simulink model "ver1_3DOF_draft2"  (R2023b)
settings: Solver=FixedStepAuto  StartTime=current_time  StopTime=40  RelTol=1e-3
values from neighbouring files (symbols this model uses):
  current_height = 0    [wrapper_for_simulink.m]
  current_pitch = 0    [wrapper_for_simulink.m]
  current_vel = 0    [wrapper_for_simulink.m]
undefined symbols (not defined in the file or in its folder): HDBK, Light, magnitude, MIL, STD
libraries: aerolibwind2 x3, aerolibasang x2, aerolibadyn x1, aerolibatmos2 x1
settings Model: Creator=User  LastModifiedBy=User
settings DataIOCC: ReturnWorkspaceOutputsName=tp3ca22a37_fc90_43f8_8ebe_8c0e39ad763e
settings DebuggingCC: AlgebraicLoopMsg=none  ArtificialAlgebraicLoopMsg=none

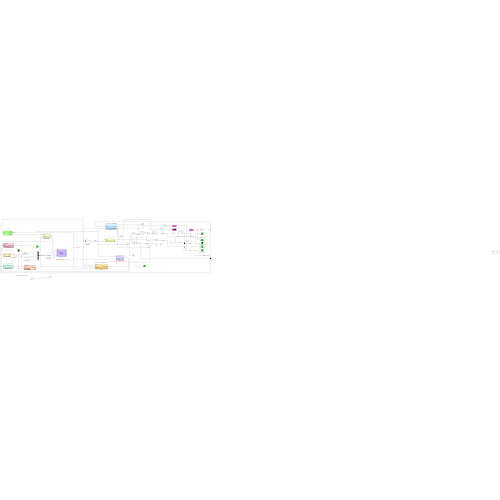
[thumbnail: Simulink's stored preview of the top-level diagram]
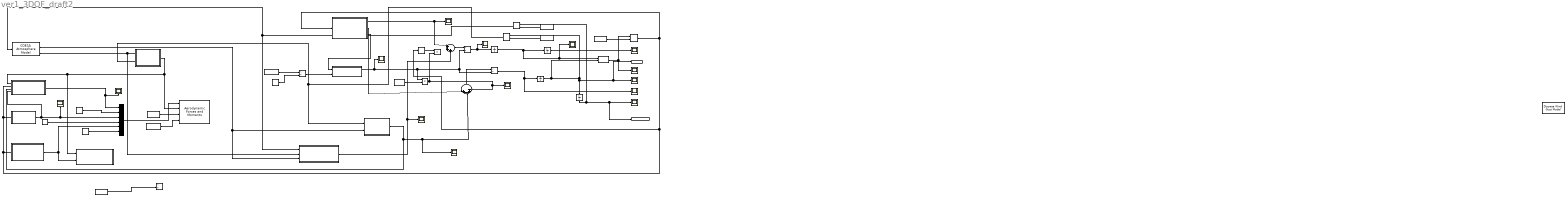
== system ver1_3DOF_draft2 ==
  note: pitch damping moment: see pg 44 of OR doc
  note: ignore everything after v = 0
  note: need to figure out how the wind parameters here
  note: why is this so high???
  note: drag is too high rn at high mach, will need to wait for better drag curve
  note: future me issue :), doesn't have much impact on the sim
      | (Take into consideration later)
  " m(t)" : Subsystem
  "Aerodynamic Forces and Moments " : aerolibadyn/Aerodynamic Forces and Moments   inputAxes=Body  outputForceAxes=Body  outputMomentAxes=Body  S=0.016513  b=2.91  cbar=0.145
  Atan2 : Trigonometry  Operator=atan2
  Axial force coefficient : Subsystem
  CG rocket : Constant  Value=[0 0 1.16]  VectorParams1D=off
  COESA Atmosphere Model : aerolibatmos2/COESA Atmosphere Model  units=Metric (MKS)  spec=MIL-STD-210C  model=Profile  profile_var=Low temperature  profile_percent=10%  profile_alt=5 km (16404 ft)  envelope_var=High temperature  envelope_percent=1%  action=Warning
  CP rocket : Constant  Value=[0 0 0.95]  VectorParams1D=off
  Delay1 : Delay  DelayLength=1  InitialConditionSource=Input port
      settings: InputPortMap=u0,p4
  Delay2 : Delay  DelayLength=1  InitialConditionSource=Input port
      settings: InputPortMap=u0,p4
  Delay3 : Delay  DelayLength=1  InitialConditionSource=Input port
      settings: InputPortMap=u0,p4
  Discrete Wind Gust Model : aerolibwind2/Discrete Wind Gust Model  units=Metric (MKS)  Gx=on  Gy=on  Gz=on  t_0=5  d_m=[120 120 80]  v_m=[3.5 3.5 3.0]
  Divide{,1..3} (4 alike) : Product  Inputs=*/
  Dynamic Pressure : Subsystem
  Flight path angle : Scope
  Integrator{,1..3} (4 alike) : Integrator
  Normal Force coefficient : Subsystem
  Pitch moment : Subsystem
  Pitch moment coefficient : Subsystem
  Product1 : Product
  Product2 : Product
  Scope{,1..8} (9 alike) : Scope
  Side force coefficient : Constant  Value=0
  Sin : Trigonometry
  Sum : Sum  Inputs=|+--+-
  Sum1 : Sum  Inputs=|+++
  Vector Concatenate : Concatenate  NumInputs=6
  WIND : Subsystem
  current height : Constant  Value=current_height
  current pitch : Constant  Value=current_pitch
  current velocity : Constant  Value=current_vel
  drag : Subsystem
  gravity g : Constant  Value=9.80665
  horizontal distance : Scope
  moi : Constant  Value=18.065
  propellant mass : Constant  Value=9.4
  roll moment coefficient : Constant  Value=0
  thrust : Subsystem
  total impulse : Constant  Value=20145.7
  vertical acceleration : Scope
  vertical height : Scope
  vertical velocity in earth ref : Scope
  yaw moment coefficient : Constant  Value=0
  Out1 : Outport  SignalName=height
  Out2 : Outport  Port=2  SignalName=velocity
  wires:
  Integrator1/1 -> Atan2/2, Integrator/1, Out2/1, vertical velocity in earth ref/1, Delay2/1  "velocity"
  CG rocket/1 -> "Aerodynamic Forces and Moments "/3
  CP rocket/1 -> "Aerodynamic Forces and Moments "/4
  COESA Atmosphere Model/2 -> WIND/3(speed of sound), drag/2(speed of sound)  "speed of sound"
  Sum/1 -> Divide1/1
  thrust/2(vertical thrust) -> Sum/1
  Delay1/1 -> Sin/1, Axial force coefficient/2(pitch angle), Normal Force coefficient/1(pitch angle), Pitch moment coefficient/1(pitch angle), thrust/1(pitch angle)
  drag/1(Drag Force) -> Axial force coefficient/3(Drag Force), Scope2/1, Sum/3
  Dynamic Pressure/1(qbar) -> "Aerodynamic Forces and Moments "/2, Pitch moment/1(dynammic pressure), Axial force coefficient/1(dynammic pressure)
  Side force coefficient/1 -> Vector Concatenate/2
  roll moment coefficient/1 -> Vector Concatenate/4
  Normal Force coefficient/1(Normal) -> Axial force coefficient/4(Normal Force coefficient), Vector Concatenate/3, Scope1/1  "Normal Force coefficient"
  Pitch moment coefficient/1(pitch moment coefficient) -> Pitch moment/2(pitch moment coefficient), Vector Concatenate/5
  yaw moment coefficient/1 -> Vector Concatenate/6
  Delay2/1 -> drag/1(velocity vector), Dynamic Pressure/2(velocity signal)
  current velocity/1 -> Delay2/2
  current height/1 -> Delay3/2
  current pitch/1 -> Delay1/2
  COESA Atmosphere Model/4 -> WIND/2(In2), Dynamic Pressure/1(Air Density)
  " m(t)"/1(m(t)) -> Scope6/1, Product1/1, Divide1/2, Divide2/2
  thrust/3(magnitude of T) -> " m(t)"/1(thrust)
  Integrator/1 -> Delay3/1, Out1/1, vertical height/1  "height"
  gravity g/1 -> Product1/2
  Vector Concatenate/1 -> "Aerodynamic Forces and Moments "/1  "aerodynamic coefficients"
  Axial force coefficient/1("axial force coefficient ") -> Scope4/1, Vector Concatenate/1
  total impulse/1 -> Divide/1
  propellant mass/1 -> Divide/2
  Divide/1 -> " m(t)"/2(exhaust velocity)
  Divide1/1 -> vertical acceleration/1, Integrator1/1  "vertical accel"
  Atan2/1 -> Delay1/1, Flight path angle/1
  Delay3/1 -> WIND/1(Altitude), COESA Atmosphere Model/1
  Sum1/1 -> Divide2/1  "Fx"
  WIND/1(wind force u direction) -> Scope3/1, Sum1/3
  Integrator2/1 -> Scope/1, Atan2/1, Integrator3/1  "horizontal vel"
  Integrator3/1 -> horizontal distance/1
  Divide2/1 -> Scope8/1, Integrator2/1  "horizontal accel"
  Product1/1 -> Scope5/1, Sum/5, Product2/2  "gravitational"
  Sin/1 -> Product2/1
  thrust/1(horizontal thrust) -> Sum1/1, Scope7/1
  moi/1 -> Divide3/2

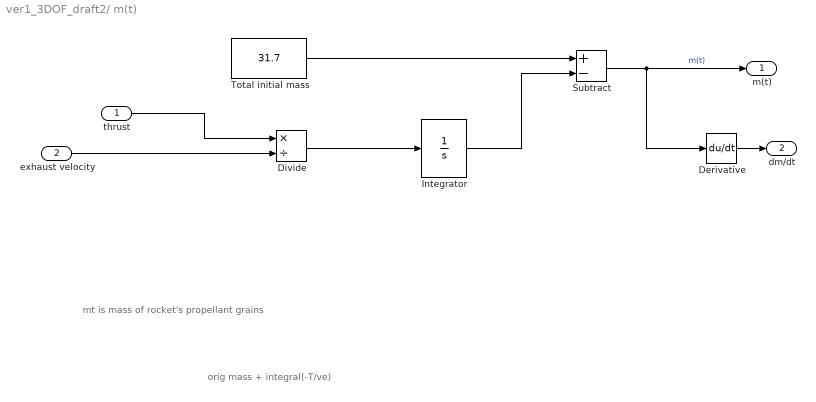
== system ver1_3DOF_draft2/ m(t) ==
  note: orig mass + integral(-T/ve)
  note: mt is mass of rocket's propellant grains
  thrust : Inport
  exhaust velocity : Inport  Port=2
  Derivative : Derivative
  Divide : Product  Inputs=*/
  Integrator : Integrator
  Subtract : Sum  Inputs=+-
  Total initial mass : Constant  Value=31.7
  m(t) : Outport
  dm/dt : Outport  Port=2
  wires:
  Total initial mass/1 -> Subtract/1
  Subtract/1 -> Derivative/1, m(t)/1  "m(t)"
  thrust/1 -> Divide/1
  exhaust velocity/1 -> Divide/2
  Divide/1 -> Integrator/1
  Integrator/1 -> Subtract/2
  Derivative/1 -> dm/dt/1

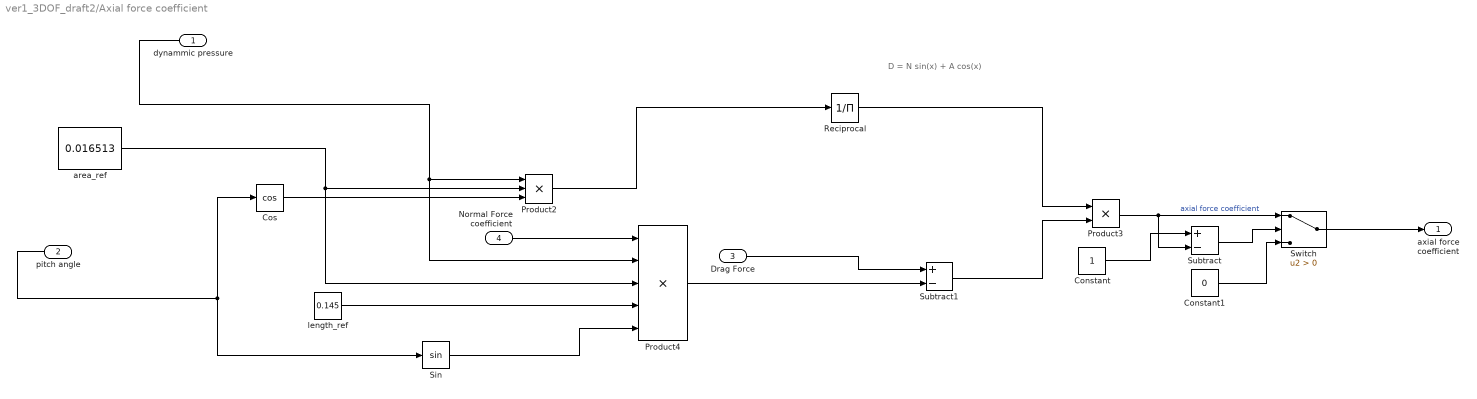
== system ver1_3DOF_draft2/Axial force coefficient ==
  note: D = N sin(x) + A cos(x)
  dynammic pressure : Inport
  pitch angle : Inport  Port=2
  Drag Force : Inport  Port=3
  Normal Force coefficient : Inport  Port=4
  Constant : Constant
  Constant1 : Constant  Value=0
  Cos : Trigonometry  Operator=cos
  Product2 : Product  Inputs=3
  Product3 : Product
  Product4 : Product  Inputs=5
  Reciprocal : Product  Inputs=/
  Sin : Trigonometry
  Subtract : Sum  Inputs=+-
  Subtract1 : Sum  Inputs=+-
  Switch : Switch  Criteria=u2 > Threshold  SaturateOnIntegerOverflow=off  InputSameDT=off
  area_ref : Constant  Value=0.016513
  length_ref : Constant  Value=0.145
  "axial force coefficient " : Outport
  wires:
  Sin/1 -> Product4/5
  pitch angle/1 -> Sin/1, Cos/1
  Normal Force coefficient/1 -> Product4/1
  dynammic pressure/1 -> Product4/2, Product2/1
  area_ref/1 -> Product2/2, Product4/3
  Cos/1 -> Product2/3
  length_ref/1 -> Product4/4
  Product4/1 -> Subtract1/2
  Product3/1 -> Subtract/2, Switch/1  "axial force coefficient"
  Subtract1/1 -> Product3/2
  Drag Force/1 -> Subtract1/1
  Product2/1 -> Reciprocal/1
  Reciprocal/1 -> Product3/1
  Switch/1 -> "axial force coefficient "/1
  Constant/1 -> Subtract/1
  Subtract/1 -> Switch/2
  Constant1/1 -> Switch/3

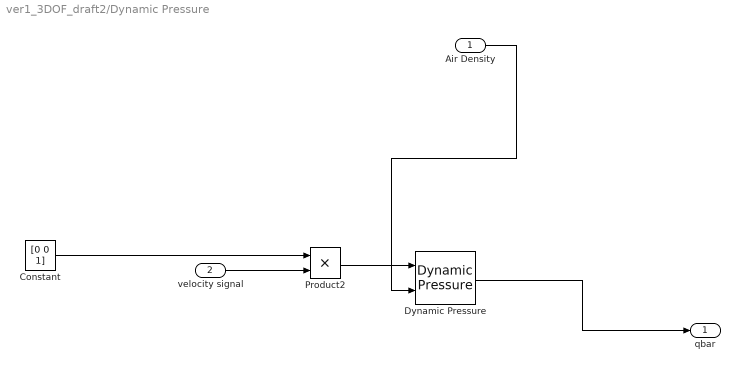
== system ver1_3DOF_draft2/Dynamic Pressure ==
  Air Density : Inport
  velocity signal : Inport  Port=2
  Constant : Constant  Value=[0 0 1]  VectorParams1D=off
  Dynamic Pressure : aerolibasang/Dynamic Pressure
  Product2 : Product
  qbar : Outport
  wires:
  Product2/1 -> Dynamic Pressure/1
  Constant/1 -> Product2/1
  Dynamic Pressure/1 -> qbar/1
  Air Density/1 -> Dynamic Pressure/2
  velocity signal/1 -> Product2/2

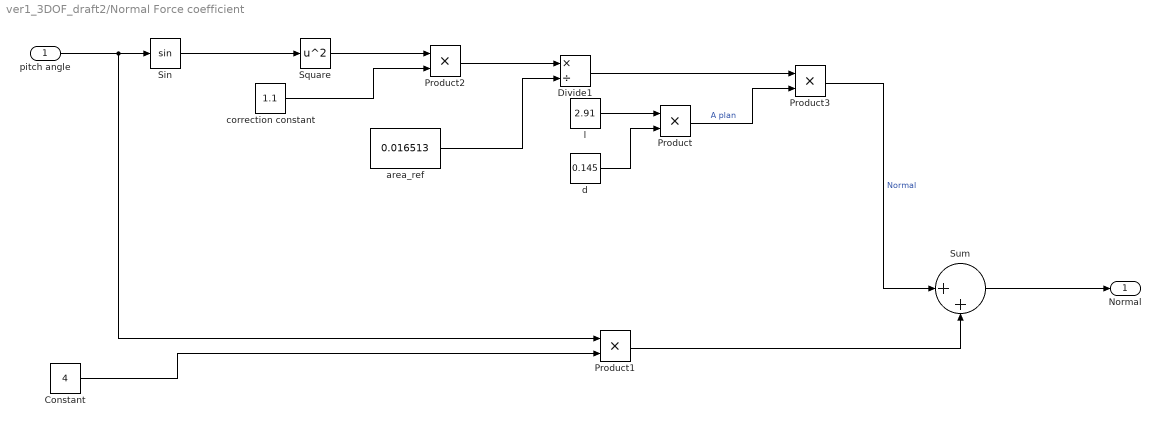
== system ver1_3DOF_draft2/Normal Force coefficient ==
  pitch angle : Inport
  Constant : Constant  Value=4
  Divide1 : Product  Inputs=*/
  Product{,1..3} (4 alike) : Product
  Sin : Trigonometry
  Square : Math  Operator=square
  Sum : Sum  Inputs=|++
  area_ref : Constant  Value=0.016513
  correction constant : Constant  Value=1.1
  d : Constant  Value=0.145
  l : Constant  Value=2.91
  Normal : Outport
  wires:
  pitch angle/1 -> Product1/1, Sin/1
  correction constant/1 -> Product2/2
  Product2/1 -> Divide1/1
  area_ref/1 -> Divide1/2
  Divide1/1 -> Product3/1
  Sin/1 -> Square/1
  Square/1 -> Product2/1
  Product/1 -> Product3/2  "A plan"
  l/1 -> Product/1
  d/1 -> Product/2
  Constant/1 -> Product1/2
  Product1/1 -> Sum/2
  Product3/1 -> Sum/1  "Normal"
  Sum/1 -> Normal/1

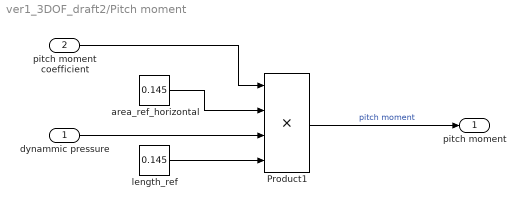
== system ver1_3DOF_draft2/Pitch moment ==
  dynammic pressure : Inport
  pitch moment coefficient : Inport  Port=2
  Product1 : Product  Inputs=4
  area_ref_horizontal : Constant  Value=0.145
  length_ref : Constant  Value=0.145
  pitch moment : Outport
  wires:
  area_ref_horizontal/1 -> Product1/2
  Product1/1 -> pitch moment/1  "pitch moment"
  length_ref/1 -> Product1/4
  dynammic pressure/1 -> Product1/3
  pitch moment coefficient/1 -> Product1/1

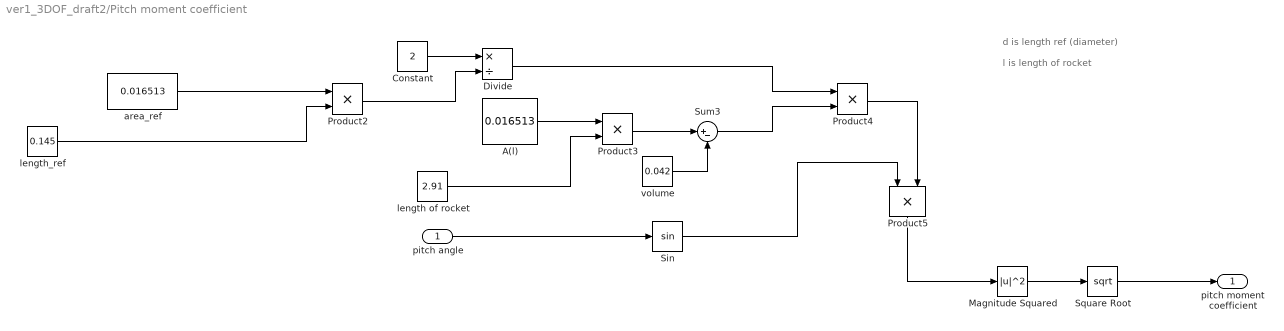
== system ver1_3DOF_draft2/Pitch moment coefficient ==
  note: l is length of rocket
  note: d is length ref (diameter)
  pitch angle : Inport
  A(l) : Constant  Value=0.016513
  Constant : Constant  Value=2
  Divide : Product  Inputs=*/
  Magnitude Squared : Math  Operator=magnitude^2
  Product{2..5} (4 alike) : Product
  Sin : Trigonometry
  Square Root : Sqrt
  Sum3 : Sum  Inputs=|+-
  area_ref : Constant  Value=0.016513
  length of rocket : Constant  Value=2.91
  length_ref : Constant  Value=0.145
  volume : Constant  Value=0.042
  pitch moment coefficient : Outport
  wires:
  length_ref/1 -> Product2/2
  Product2/1 -> Divide/2
  A(l)/1 -> Product3/1
  Product4/1 -> Product5/2
  Product5/1 -> Magnitude Squared/1
  area_ref/1 -> Product2/1
  Product3/1 -> Sum3/1
  Divide/1 -> Product4/1
  volume/1 -> Sum3/2
  Constant/1 -> Divide/1
  pitch angle/1 -> Sin/1
  Sum3/1 -> Product4/2
  Sin/1 -> Product5/1
  length of rocket/1 -> Product3/2
  Magnitude Squared/1 -> Square Root/1
  Square Root/1 -> pitch moment coefficient/1

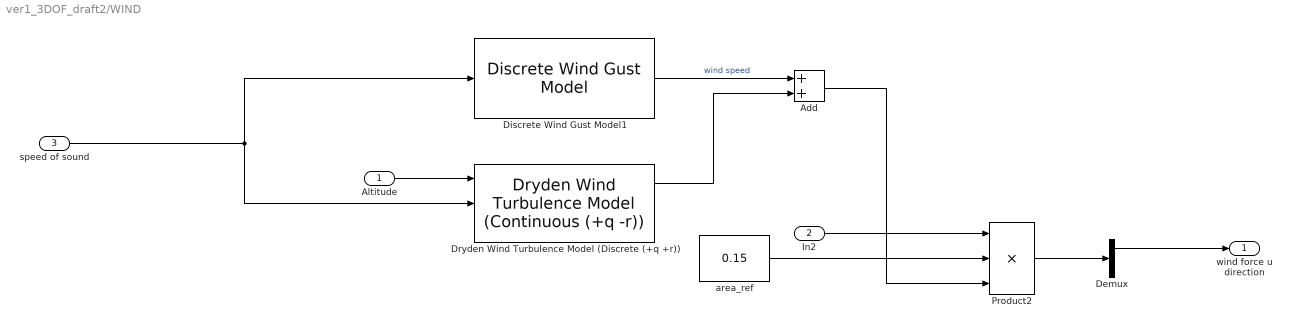
== system ver1_3DOF_draft2/WIND ==
  Altitude : Inport
  In2 : Inport  Port=2
  speed of sound : Inport  Port=3
  Add : Sum
  Demux : Demux  Outputs=3
  Discrete Wind Gust Model1 : aerolibwind2/Discrete Wind Gust Model  units=Metric (MKS)  Gx=on  Gy=on  Gz=on  t_0=0  d_m=[50 80 50]  v_m=[1 2 3.0]
  Dryden Wind Turbulence Model (Discrete (+q +r)) : aerolibwind2/Dryden Wind Turbulence Model  (Continuous (+q -r))  units=Metric (MKS)  spec=MIL-HDBK-1797B  model=Discrete Dryden (+q +r)  W20=5  Wdeg=10  TurbProb=10^-2 - Light  L_high=533.4  Wingspan=10  ts=0.1  Seed=[23341 23342 23343 23344]  T_on=on
      settings: LibrarySourceBlock=|
      | aerolibwind2/Dryden Wind Turbulence Model
      | (Discrete (+q +r))
  Product2 : Product  Inputs=3
  area_ref : Constant  Value=0.15
  wind force u direction : Outport
  wires:
  In2/1 -> Product2/1
  area_ref/1 -> Product2/2
  Dryden Wind Turbulence Model (Discrete (+q +r))/1 -> Add/2
  speed of sound/1 -> Discrete Wind Gust Model1/1, Dryden Wind Turbulence Model (Discrete (+q +r))/2
  Product2/1 -> Demux/1
  Altitude/1 -> Dryden Wind Turbulence Model (Discrete (+q +r))/1
  Discrete Wind Gust Model1/1 -> Add/1  "wind speed"
  Add/1 -> Product2/3
  Demux/1 -> wind force u direction/1

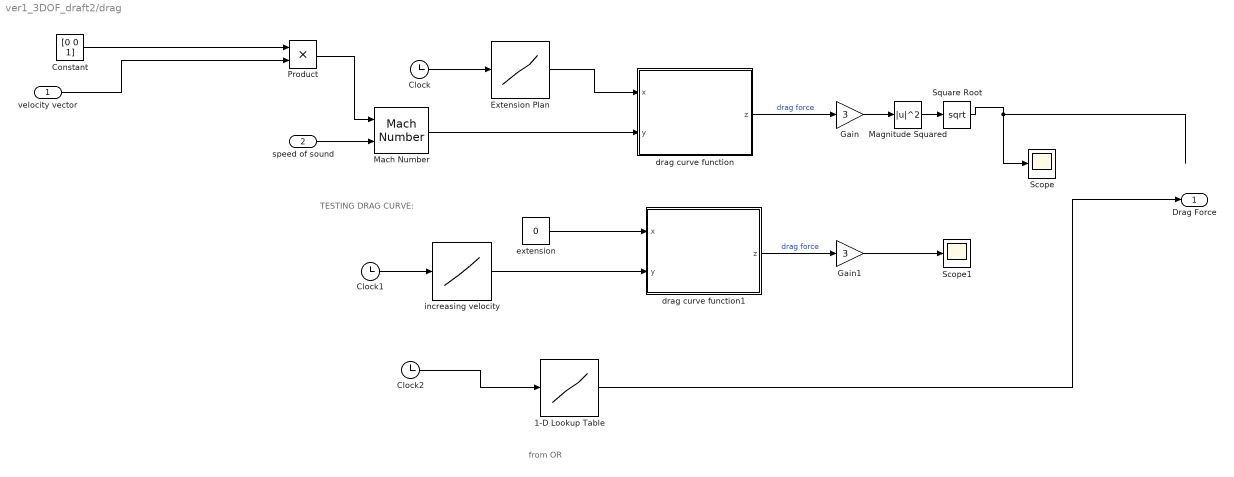
== system ver1_3DOF_draft2/drag ==
  note: from OR
  note: TESTING DRAG CURVE:
  velocity vector : Inport
  speed of sound : Inport  Port=2
  1-D Lookup Table : Lookup_n-D  NumberOfTableDimensions=1  BreakpointsForDimension1=|  Table=|  InternalRulePriority=Speed  RndMeth=Simplest
      BreakpointsForDimension1=|
      | [0.01
      | 0.02
      | 0.03
      | 0.04
      | 0.05
      | 0.06
      | 0.07
      | 0.078
      | 0.085
      | 0.092
      | 0.098
      | 0.104
      | 0.109
      | 0.114
      | 0.121
      | 0.133
      | 0.15
      | 0.175
      | 0.213
      | 0.263
      | 0.313
      | 0.363
      | 0.413
      | 0.463
      | 0.513
      | 0.563
      | 0.613
      | 0.663
      | 0.713
      | 0.763
      | 0.813
      | 0.863
      | 0.913
      | 0.963
      | 1.013
      | 1.063
      | 1.113
      | 1.163
      | 1.213
      | 1.263
      | 1.313
      | 1.363
      | 1.413
      | 1.463
      | 1.513
      | 1.563
      | 1.613
      | 1.663
      | 1.713
      | 1.763
      | 1.813
      | 1.863
      | 1.913
      | 1.963
      | 2.013
      | 2.063
      | 2.113
      | 2.163
      | 2.213
      | 2.263
      | 2.313
      | 2.363
      | 2.413
      | 2.463
      | 2.513
      | 2.563
      | 2.613
      | 2.663
      | 2.713
      | 2.763
      | 2.813
      | 2.863
      | 2.913
      | 2.963
      | 3.013
      | 3.063
      | 3.113
      | 3.163
      | 3.213
      | 3.263
      | 3.313
      | 3.363
      | 3.413
      | 3.463
      | 3.513
      | 3.563
      | 3.594
      | 3.64
      | 3.69
      | 3.74
      | 3.79
      | 3.84
      | 3.89
      | 3.94
      | 3.99
      | 4.04
      | 4.09
      | 4.14
      | 4.19
      | 4.24
      | 4.29
      | 4.34
      | 4.39
      | 4.44
      | 4.49
      | 4.54
      | 4.59
      | 4.64
      | 4.69
      | 4.74
      | 4.79
      | 4.84
      | 4.89
      | 4.94
      | 4.99
      | 5.04
      | 5.09
      | 5.14
      | 5.19
      | 5.24
      | 5.29
      | 5.34
      | 5.39
      | 5.44
      | 5.49
      | 5.54
      | 5.59
      | 5.64
      | 5.69
      | 5.74
      | 5.79
      | 5.84
      | 5.89
      | 5.94
      | 5.99
      | 6.04
      | 6.09
      | 6.14
      | 6.19
      | 6.24
      | 6.29
      | 6.34
      | 6.39
      | 6.44
      | 6.49
      | 6.54
      | 6.59
      | 6.64
      | 6.69
      | 6.74
      | 6.79
      | 6.84
      | 6.89
      | 6.94
      | 6.99
      | 7.04
      | 7.09
      | 7.14
      | 7.19
      | 7.24
      | 7.29
      | 7.34
      | 7.39
      | 7.44
      | 7.49
      | 7.54
      | 7.59
      | 7.64
      | 7.69
      | 7.74
      | 7.79
      | 7.84
      | 7.89
      | 7.94
      | 7.99
      | 8.04
      | 8.09
      | 8.14
      | 8.19
      | 8.24
      | 8.29
      | 8.34
      | 8.39
      | 8.44
      | 8.49
      | 8.54
      | 8.59
      | 8.64
      | 8.69
      | 8.74
      | 8.79
      | 8.84
      | 8.89
      | 8.94
      | 8.99
      | 9.04
      | 9.09
      | 9.14
      | 9.19
      | 9.24
      | 9.29
      | 9.34
      | 9.39
      | 9.44
      | 9.49
      | 9.54
      | 9.59
      | 9.64
      | 9.69
      | 9.74
      | 9.79
      | 9.84
      | 9.89
      | 9.94
      | 9.99
      | 10.04
      | 10.09
      | 10.14
      | 10.19
      | 10.24
      | 10.29
      | 10.34
      | 10.39
      | 10.44
      | 10.49
      | 10.54
      | 10.59
      | 10.64
      | 10.69
      | 10.74
      | 10.79
      | 10.84
      | 10.89
      | 10.94
      | 10.99
      | 11.04
      | 11.09
      | 11.14
      | 11.19
      | 11.24
      | 11.29
      | 11.34
      | 11.39
      | 11.44
      | 11.49
      | 11.54
      | 11.59
      | 11.64
      | 11.69
      | 11.74
      | 11.79
      | 11.84
      | 11.89
      | 11.94
      | 11.99
      | 12.04
      | 12.09
      | 12.14
      | 12.19
      | 12.24
      | 12.29
      | 12.34
      | 12.39
      | 12.44
      | 12.49
      | 12.54
      | 12.59
      | 12.64
      | 12.69
      | 12.74
      | 12.79
      | 12.84
      | 12.89
      | 12.94
      | 12.99
      | 13.04
      | 13.09
      | 13.14
      | 13.19
      | 13.24
      | 13.29
      | 13.34
      | 13.39
      | 13.44
      | 13.49
      | 13.54
      | 13.59
      | 13.64
      | 13.69
      | 13.74
      | 13.79
      | 13.84
      | 13.89
      | 13.94
      | 13.99
      | 14.04
      | 14.09
      | 14.14
      | 14.19
      | 14.24
      | 14.29
      | 14.34
      | 14.39
      | 14.44
      | 14.49
      | 14.54
      | 14.59
      | 14.64
      | 14.69
      | 14.74
      | 14.79
      | 14.84
      | 14.89
      | 14.94
      | 14.99
      | 15.04
      | 15.09
      | 15.14
      | 15.19
      | 15.24
      | 15.29
      | 15.34
      | 15.39
      | 15.44
      | 15.49
      | 15.54
      | 15.59
      | 15.64
      | 15.69
      | 15.74
      | 15.79
      | 15.84
      | 15.89
      | 15.94
      | 15.99
      | 16.04
      | 16.09
      | 16.14
      | 16.19
      | 16.24
      | 16.29
      | 16.34
      | 16.39
      | 16.44
      | 16.49
      | 16.54
      | 16.59
      | 16.64
      | 16.69
      | 16.74
      | 16.79
      | 16.84
      | 16.89
      | 16.94
      | 16.99
      | 17.04
      | 17.09
      | 17.14
      | 17.19
      | 17.24
      | 17.29
      | 17.34
      | 17.39
      | 17.44
      | 17.49
      | 17.54
      | 17.59
      | 17.64
      | 17.69
      | 17.74
      | 17.79
      | 17.84
      | 17.89
      | 17.94
      | 17.99
      | 18.04
      | 18.09
      | 18.14
      | 18.19
      | 18.24
      | 18.29
      | 18.34
      | 18.39
      | 18.44
      | 18.49
      | 18.54
      | 18.59
      | 18.64
      | 18.69
      | 18.74
      | 18.79
      | 18.84
      | 18.89
      | 18.94
      | 18.99
      | 19.04
      | 19.09
      | 19.14
      | 19.19
      | 19.24
      | 19.29
      | 19.34
      | 19.39
      | 19.44
      | 19.49
      | 19.54
      | 19.59
      | 19.64
      | 19.69
      | 19.74
      | 19.79
      | 19.84
      | 19.89
      | 19.94
      | 19.99
      | 20.04
      | 20.09
      | 20.14
      | 20.19
      | 20.24
      | 20.29
      | 20.34
      | 20.39
      | 20.44
      | 20.49
      | 20.54
      | 20.59
      | 20.64
      | 20.69
      | 20.74
      | 20.79
      | 20.84
      | 20.89
      | 20.94
      | 20.99
      | 21.04
      | 21.09
      | 21.14
      | 21.19
      | 21.24
      | 21.29
      | 21.34
      | 21.39
      | 21.44
      | 21.49
      | 21.54
      | 21.59
      | 21.64
      | 21.69
      | 21.74
      | 21.79
      | 21.84
      | 21.89
      | 21.94
      | 21.99
      | 22.04
      | 22.09
      | 22.14
      | 22.19
      | 22.24
      | 22.29
      | 22.34
      | 22.39
      | 22.44
      | 22.49
      | 22.54
      | 22.59
      | 22.64
      | 22.69
      | 22.74
      | 22.79
      | 22.84
      | 22.89
      | 22.94
      | 22.99
      | 23.04
      | 23.09
      | 23.14
      | 23.19
      | 23.24
      | 23.29
      | 23.34
      | 23.39
      | 23.44
      | 23.49
      | 23.54
      | 23.59
      | 23.64
      | 23.69
      | 23.74
      | 23.79
      | 23.84
      | 23.89
      | 23.94
      | 23.99
      | 24.04
      | 24.09
      | 24.14
      | 24.19
      | 24.24
      | 24.29
      | 24.34
      | 24.39
      | 24.44
      | 24.49
      | 24.54
      | 24.59
      | 24.64
      | 24.69
      | 24.74
      | 24.79
      | 24.84
      | 24.89
      | 24.94
      | 24.99
      | 25.04
      | 25.09
      | 25.14
      | 25.19
      | 25.24
      | 25.29
      | 25.34
      | 25.39
      | 25.44
      | 25.49
      | 25.54
      | 25.59
      | 25.64
      | 25.69
      | 25.74
      | 25.79
      | 25.84
      | 25.89
      | 25.94
      | 25.99
      | 26.04
      | 26.09
      | 26.14
      | 26.19
      | 26.24
      | 26.29
      | 26.34
      | 26.39
      | 26.44
      | 26.49
      | 26.54
      | 26.59
      | 26.64
      | 26.69
      | 26.74
      | 26.79
      | 26.84
      | 26.89
      | 26.94
      | 26.99
      | 27.04
      | 27.09
      | 27.14
      | 27.19
      | 27.24
      | 27.29
      | 27.34
      | 27.39
      | 27.44
      | 27.49
      | 27.54
      | 27.59
      | 27.64
      | 27.69
      | 27.74
      | 27.79
      | 27.84
      | 27.89
      | 27.94
      | 27.99
      | 28.04
      | 28.09
      | 28.14
      | 28.19
      | 28.24
      | 28.29
      | 28.34
      | 28.39
      | 28.44
      | 28.49
      | 28.54
      | 28.59
      | 28.64
      | 28.69
      | 28.74
      | 28.79
      | 28.84
      | 28.89
      | 28.94
      | 28.99
      | 29.04
      | 29.09
      | 29.14
      | 29.19
      | 29.24
      | 29.29
      | 29.34
      | 29.39
      | 29.44
      | 29.49
      | 29.54
      | 29.59
      | 29.64
      | 29.69
      | 29.74
      | 29.79
      | 29.84
      | 29.89
      | 29.94
      | 29.99
      | 30.04
      | 30.09
      | 30.14
      | 30.19
      | 30.24
      | 30.29
      | 30.34
      | 30.39
      | 30.44
      | 30.49
      | 30.54
      | 30.59
      | 30.64
      | 30.69
      | 30.74
      | 30.79
      | 30.84
      | 30.89
      | 30.94
      | 30.99
      | 31.04
      | 31.09
      | 31.14
      | 31.19
      | 31.24
      | 31.29
      | 31.34
      | 31.39
      | 31.44
      | 31.49
      | 31.54
      | 31.59
      | 31.64
      | 31.69
      | 31.74
      | 31.79
      | 31.84
      | 31.89
      | 31.94
      | 31.99
      | 32.04
      | 32.09
      | 32.14
      | 32.19
      | 32.24
      | 32.29
      | 32.34
      | 32.39
      | 32.44
      | 32.49
      | 32.54
      | 32.59
      | 32.64
      | 32.69
      | 32.74
      | 32.79
      | 32.84
      | 32.89
      | 32.94
      | 32.99
      | 33.04
      | 33.09
      | 33.14
      | 33.19
      | 33.24
      | 33.29
      | 33.34
      | 33.39
      | 33.44
      | 33.49
      | 33.54
      | 33.59
      | 33.64
      | 33.69
      | 33.74
      | 33.79
      | 33.84
      | 33.89
      | 33.94
      | 33.99
      | 34.04
      | 34.09
      | 34.14
      | 34.19
      | 34.24
      | 34.29
      | 34.34
      | 34.39
      | 34.44
      | 34.49
      | 34.54
      | 34.59
      | 34.64
      | 34.69
      | 34.74
      | 34.79
      | 34.84
      | 34.89
      | 34.94
      | 34.99
      | 35.04
      | 35.09
      | 35.14
      | 35.19
      | 35.24
      | 35.29
      | 35.34
      | 35.39
      | 35.44
      | 35.49
      | 35.54
      | 35.59
      | 35.64
      | 35.69
      | 35.74
      | 35.79
      | 35.84
      | 35.89
      | 35.94
      | 35.99
      | 36.04
      | 36.09
      | 36.14
      | 36.19
      | 36.24
      | 36.29
      | 36.34
      | 36.39
      | 36.44
      | 36.49
      | 36.54
      | 36.59
      | 36.64
      | 36.69
      | 36.74
      | 36.79
      | 36.84
      | 36.89
      | 36.94
      | 36.99
      | 37.04
      | 37.09
      | 37.14
      | 37.19
      | 37.24
      | 37.29
      | 37.34
      | 37.39
      | 37.44
      | 37.49
      | 37.54
      | 37.59
      | 37.64
      | 37.69
      | 37.74
      | 37.79
      | 37.84
      | 37.89
      | 37.94
      | 37.99
      | 38.04
      | 38.09
      | 38.14
      | 38.19
      | 38.24
      | 38.29
      | 38.34
      | 38.39
      | 38.44
      | 38.49
      | 38.54
      | 38.59]
      Table=|
      | [6.45E-04
      | 0.027
      | 0.105
      | 0.212
      | 0.338
      | 0.481
      | 0.642
      | 0.809
      | 0.971
      | 1.131
      | 1.288
      | 1.444
      | 1.597
      | 1.75
      | 1.994
      | 2.391
      | 3.057
      | 4.223
      | 6.343
      | 9.812
      | 14.076
      | 19.157
      | 25.083
      | 31.887
      | 39.581
      | 48.209
      | 57.793
      | 68.372
      | 79.961
      | 92.62
      | 106.378
      | 121.275
      | 137.345
      | 154.63
      | 173.191
      | 193.08
      | 214.392
      | 237.207
      | 261.655
      | 287.921
      | 316.302
      | 347.256
      | 381.815
      | 409.873
      | 439.455
      | 471.847
      | 504.945
      | 536.656
      | 566.911
      | 596.248
      | 625.958
      | 655.947
      | 685.233
      | 714.695
      | 744.391
      | 774.108
      | 803.758
      | 833.016
      | 860.081
      | 886.859
      | 913.355
      | 939.504
      | 965.311
      | 990.775
      | 1014.79
      | 1038.216
      | 1061.179
      | 1083.078
      | 1102.884
      | 1120.561
      | 1136.108
      | 1149.568
      | 1160.938
      | 1170.235
      | 1177.488
      | 1183.267
      | 1188.088
      | 1191.815
      | 1194.392
      | 1195.121
      | 1193.871
      | 1190.726
      | 1185.86
      | 1179.236
      | 1170.729
      | 1161.001
      | 1154.569
      | 1144.059
      | 1132.871
      | 1121.805
      | 1110.852
      | 1100.033
      | 1089.521
      | 1079.134
      | 1068.852
      | 1058.678
      | 1048.611
      | 1038.652
      | 1028.805
      | 1019.068
      | 1009.423
      | 999.893
      | 990.463
      | 981.13
      | 971.899
      | 962.759
      | 953.729
      | 944.789
      | 936.004
      | 927.416
      | 918.919
      | 910.506
      | 902.172
      | 893.931
      | 885.777
      | 877.709
      | 869.72
      | 861.81
      | 853.975
      | 846.226
      | 838.567
      | 830.976
      | 823.465
      | 816.03
      | 808.672
      | 801.382
      | 794.212
      | 787.142
      | 780.028
      | 772.982
      | 766.011
      | 759.116
      | 752.29
      | 745.536
      | 738.855
      | 732.245
      | 725.699
      | 719.217
      | 712.807
      | 706.464
      | 700.185
      | 693.969
      | 687.816
      | 681.728
      | 675.707
      | 669.741
      | 663.905
      | 658.167
      | 652.486
      | 646.859
      | 641.282
      | 635.764
      | 630.3
      | 624.9
      | 619.544
      | 614.241
      | 608.992
      | 603.795
      | 598.657
      | 593.556
      | 588.512
      | 583.512
      | 578.552
      | 573.386
      | 568.273
      | 563.228
      | 558.231
      | 553.307
      | 548.495
      | 543.737
      | 539.025
      | 534.355
      | 529.743
      | 525.18
      | 520.658
      | 516.186
      | 511.757
      | 507.373
      | 503.037
      | 498.737
      | 494.486
      | 490.28
      | 486.111
      | 481.99
      | 477.91
      | 473.87
      | 469.865
      | 465.9
      | 461.977
      | 458.095
      | 454.242
      | 450.495
      | 446.792
      | 443.123
      | 439.484
      | 435.88
      | 432.31
      | 428.774
      | 425.278
      | 421.811
      | 418.376
      | 414.978
      | 411.607
      | 408.266
      | 404.96
      | 401.686
      | 398.438
      | 395.184
      | 391.917
      | 388.683
      | 385.479
      | 382.304
      | 379.158
      | 376.043
      | 372.957
      | 369.901
      | 366.91
      | 363.969
      | 361.048
      | 358.157
      | 355.291
      | 352.456
      | 349.644
      | 346.855
      | 344.099
      | 341.36
      | 338.65
      | 335.964
      | 333.299
      | 330.664
      | 328.054
      | 325.462
      | 322.895
      | 320.352
      | 317.766
      | 315.18
      | 312.617
      | 310.086
      | 307.575
      | 305.085
      | 302.62
      | 300.182
      | 297.762
      | 295.361
      | 293.009
      | 290.699
      | 288.411
      | 286.136
      | 283.879
      | 281.404
      | 278.963
      | 276.543
      | 274.146
      | 271.777
      | 269.437
      | 267.117
      | 264.818
      | 262.54
      | 260.293
      | 258.067
      | 255.864
      | 253.687
      | 251.525
      | 249.382
      | 247.257
      | 245.137
      | 243.044
      | 240.967
      | 238.91
      | 236.877
      | 234.858
      | 232.864
      | 230.889
      | 228.934
      | 226.999
      | 225.106
      | 223.231
      | 221.377
      | 219.541
      | 217.72
      | 215.922
      | 214.198
      | 212.551
      | 210.914
      | 209.292
      | 207.686
      | 206.089
      | 204.505
      | 202.933
      | 201.376
      | 199.835
      | 198.309
      | 196.789
      | 195.285
      | 193.788
      | 192.312
      | 190.846
      | 189.391
      | 187.954
      | 186.284
      | 184.481
      | 182.702
      | 180.957
      | 179.237
      | 177.545
      | 175.875
      | 174.234
      | 172.617
      | 171.026
      | 169.463
      | 167.925
      | 166.408
      | 164.911
      | 163.434
      | 161.976
      | 160.536
      | 159.122
      | 157.722
      | 156.33
      | 154.958
      | 153.603
      | 152.265
      | 150.943
      | 149.637
      | 148.347
      | 147.07
      | 145.809
      | 144.563
      | 143.324
      | 142.099
      | 140.889
      | 139.693
      | 138.51
      | 137.334
      | 136.173
      | 135.023
      | 133.888
      | 132.766
      | 131.657
      | 130.547
      | 129.451
      | 128.372
      | 127.304
      | 126.247
      | 125.195
      | 124.154
      | 123.123
      | 122.107
      | 121.11
      | 120.118
      | 119.136
      | 118.163
      | 117.203
      | 116.246
      | 115.3
      | 114.362
      | 113.435
      | 112.522
      | 111.61
      | 110.707
      | 109.809
      | 108.922
      | 108.045
      | 107.17
      | 106.301
      | 105.443
      | 104.597
      | 103.758
      | 102.918
      | 102.086
      | 101.264
      | 100.452
      | 99.642
      | 98.838
      | 98.046
      | 97.256
      | 96.473
      | 95.697
      | 94.928
      | 94.165
      | 93.408
      | 92.662
      | 91.919
      | 91.176
      | 90.447
      | 89.722
      | 89.003
      | 88.288
      | 87.583
      | 86.88
      | 86.184
      | 85.501
      | 84.824
      | 84.15
      | 83.482
      | 82.819
      | 82.159
      | 81.506
      | 80.86
      | 80.218
      | 79.582
      | 78.951
      | 78.32
      | 77.699
      | 77.079
      | 76.464
      | 75.853
      | 75.25
      | 74.651
      | 74.056
      | 73.465
      | 72.878
      | 72.295
      | 71.719
      | 71.145
      | 70.579
      | 70.018
      | 69.456
      | 68.898
      | 68.348
      | 67.798
      | 67.254
      | 66.718
      | 66.181
      | 65.651
      | 65.123
      | 64.6
      | 64.081
      | 63.566
      | 63.053
      | 62.543
      | 62.038
      | 61.539
      | 61.04
      | 60.547
      | 60.056
      | 59.569
      | 59.088
      | 58.608
      | 58.128
      | 57.659
      | 57.189
      | 56.726
      | 56.269
      | 55.815
      | 55.364
      | 54.915
      | 54.468
      | 54.027
      | 53.587
      | 53.151
      | 52.718
      | 52.29
      | 51.863
      | 51.437
      | 51.015
      | 50.595
      | 50.185
      | 49.77
      | 49.362
      | 48.956
      | 48.555
      | 48.153
      | 47.757
      | 47.361
      | 46.968
      | 46.578
      | 46.191
      | 45.809
      | 45.427
      | 45.048
      | 44.672
      | 44.297
      | 43.926
      | 43.557
      | 43.192
      | 42.828
      | 42.466
      | 42.106
      | 41.747
      | 41.393
      | 41.042
      | 40.692
      | 40.346
      | 40.003
      | 39.661
      | 39.32
      | 38.983
      | 38.65
      | 38.318
      | 37.985
      | 37.658
      | 37.334
      | 37.01
      | 36.689
      | 36.372
      | 36.057
      | 35.741
      | 35.429
      | 35.119
      | 34.812
      | 34.507
      | 34.203
      | 33.903
      | 33.606
      | 33.31
      | 33.015
      | 32.723
      | 32.434
      | 32.145
      | 31.858
      | 31.576
      | 31.294
      | 31.017
      | 30.744
      | 30.468
      | 30.196
      | 29.922
      | 29.648
      | 29.377
      | 29.107
      | 28.842
      | 28.579
      | 28.318
      | 28.059
      | 27.801
      | 27.544
      | 27.29
      | 27.038
      | 26.786
      | 26.537
      | 26.289
      | 26.045
      | 25.804
      | 25.562
      | 25.323
      | 25.084
      | 24.849
      | 24.616
      | 24.381
      | 24.147
      | 23.917
      | 23.689
      | 23.459
      | 23.236
      | 23.01
      | 22.787
      | 22.564
      | 22.344
      | 22.128
      | 21.912
      | 21.697
      | 21.483
      | 21.271
      | 21.061
      | 20.851
      | 20.642
      | 20.435
      | 20.228
      | 20.022
      | 19.817
      | 19.614
      | 19.412
      | 19.211
      | 19.013
      | 18.814
      | 18.619
      | 18.428
      | 18.239
      | 18.052
      | 17.866
      | 17.681
      | 17.496
      | 17.315
      | 17.13
      | 16.946
      | 16.768
      | 16.588
      | 16.406
      | 16.225
      | 16.05
      | 15.875
      | 15.699
      | 15.526
      | 15.353
      | 15.185
      | 15.017
      | 14.852
      | 14.689
      | 14.527
      | 14.366
      | 14.206
      | 14.046
      | 13.887
      | 13.73
      | 13.573
      | 13.417
      | 13.262
      | 13.107
      | 12.955
      | 12.802
      | 12.651
      | 12.501
      | 12.351
      | 12.203
      | 12.057
      | 11.911
      | 11.766
      | 11.623
      | 11.484
      | 11.344
      | 11.205
      | 11.065
      | 10.929
      | 10.794
      | 10.656
      | 10.524
      | 10.393
      | 10.26
      | 10.128
      | 9.996
      | 9.867
      | 9.737
      | 9.609
      | 9.486
      | 9.361
      | 9.241
      | 9.116
      | 8.995
      | 8.874
      | 8.757
      | 8.636
      | 8.516
      | 8.397
      | 8.281
      | 8.165
      | 8.052
      | 7.938
      | 7.826
      | 7.715
      | 7.604
      | 7.496
      | 7.388
      | 7.281
      | 7.176
      | 7.071
      | 6.966
      | 6.863
      | 6.759
      | 6.657
      | 6.555
      | 6.455
      | 6.356
      | 6.257
      | 6.159
      | 6.062
      | 5.967
      | 5.871
      | 5.776
      | 5.683
      | 5.59
      | 5.498
      | 5.407
      | 5.317
      | 5.228
      | 5.142
      | 5.053
      | 4.967
      | 4.88
      | 4.794
      | 4.711
      | 4.627
      | 4.544
      | 4.463
      | 4.381
      | 4.304
      | 4.224
      | 4.147
      | 4.073
      | 3.994
      | 3.917
      | 3.846
      | 3.77
      | 3.698
      | 3.622
      | 3.548
      | 3.481
      | 3.413
      | 3.344
      | 3.274
      | 3.209
      | 3.143
      | 3.079
      | 3.018
      | 2.949
      | 2.886
      | 2.82
      | 2.755
      | 2.691
      | 2.628
      | 2.567
      | 2.51
      | 2.45
      | 2.393
      | 2.334
      | 2.277
      | 2.222
      | 2.167
      | 2.114
      | 2.061
      | 2.009
      | 1.955
      | 1.903
      | 1.852
      | 1.803
      | 1.754
      | 1.703
      | 1.653
      | 1.605
      | 1.561
      | 1.514
      | 1.468
      | 1.424
      | 1.38
      | 1.336
      | 1.296
      | 1.254
      | 1.213
      | 1.173
      | 1.133
      | 1.094
      | 1.057
      | 1.021
      | 0.986
      | 0.953
      | 0.919
      | 0.886
      | 0.858
      | 0.829
      | 0.8
      | 0.772
      | 0.745
      | 0.713
      | 0.685
      | 0.659
      | 0.635
      | 0.611
      | 0.59
      | 0.57
      | 0.546
      | 0.52
      | 0.498
      | 0.477
      | 0.457
      | 0.438
      | 0.418
      | 0.398
      | 0.376
      | 0.361
      | 0.351
      | 0.339
      | 0.329
      | 0.311
      | 0.291
      | 0.28
      | 0.266
      | 0.247
      | 0.235
      | 0.224
      | 0.209
      | 0.191
      | 0.174
      | 0.161
      | 0.145
      | 0.13
      | 0.116
      | 0.103
      | 0.089
      | 0.076
      | 0.063
      | 0.052
      | 0.041
      | 0.03
      | 0.022
      | 0.015
      | 0.009
      | 0.005]
  Clock : Clock
  Clock1 : Clock
  Clock2 : Clock
  Constant : Constant  Value=[0 0 1]  VectorParams1D=off
  Extension Plan : Lookup_n-D  NumberOfTableDimensions=1  BreakpointsForDimension1=|  Table=|  InternalRulePriority=Speed  RndMeth=Simplest
      BreakpointsForDimension1=|
      | [0
      | 1
      | 2
      | 3
      | 4
      | 5
      | 6
      | 7
      | 8
      | 9
      | 10
      | 11
      | 12
      | 13
      | 14
      | 15
      | 16
      | 17
      | 18
      | 19
      | 20]
      Table=|
      | [0
      | 0
      | 0
      | 0
      | 0.01
      | 0.01
      | 0.01
      | 0.01
      | 0.01
      | 0
      | 0
      | 0
      | 0
      | 0
      | 0
      | 0
      | 0
      | 0
      | 0
      | 0
      | 0]
  Gain : Gain  Gain=3
  Gain1 : Gain  Gain=3
  Mach Number : aerolibasang/Mach Number
  Magnitude Squared : Math  Operator=magnitude^2
  Product : Product
  Scope : Scope
  Scope1 : Scope
  Square Root : Sqrt
  drag curve function : MATLAB Function  TreatAsAtomicUnit=on
  drag curve function1 : MATLAB Function  TreatAsAtomicUnit=on
  extension : Constant  Value=0
  increasing velocity : Lookup_n-D  NumberOfTableDimensions=1  BreakpointsForDimension1=[0 1 2 3 4 5 6 7]  Table=[0 0.1 0.2 0.3 0.4 0.5 0.6 0.7]  InternalRulePriority=Speed  RndMeth=Simplest
  Drag Force : Outport
  wires:
  drag curve function/1(z) -> Gain/1  "drag force"
  Mach Number/1 -> drag curve function/2(y)
  speed of sound/1 -> Mach Number/2
  Constant/1 -> Product/1
  Product/1 -> Mach Number/1
  velocity vector/1 -> Product/2
  Gain/1 -> Magnitude Squared/1
  Clock/1 -> Extension Plan/1
  Extension Plan/1 -> drag curve function/1(x)
  Clock1/1 -> increasing velocity/1
  extension/1 -> drag curve function1/1(x)
  drag curve function1/1(z) -> Gain1/1  "drag force"
  increasing velocity/1 -> drag curve function1/2(y)
  Gain1/1 -> Scope1/1
  Magnitude Squared/1 -> Square Root/1
  Square Root/1 -> Scope/1
  Clock2/1 -> 1-D Lookup Table/1
  1-D Lookup Table/1 -> Drag Force/1

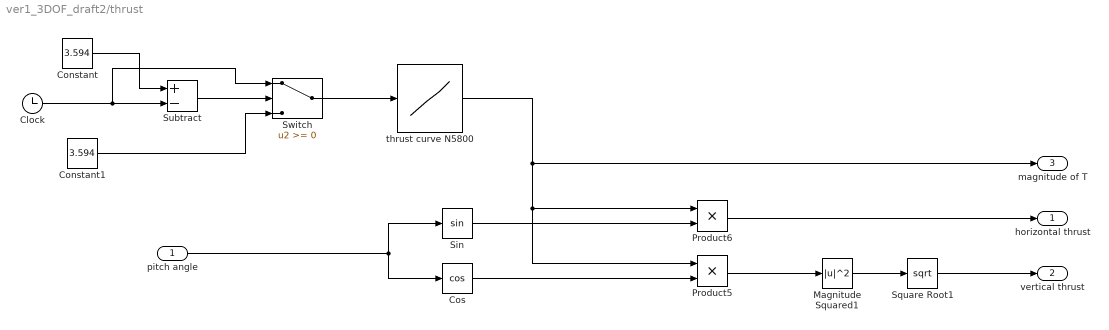
== system ver1_3DOF_draft2/thrust ==
  pitch angle : Inport
  Clock : Clock
  Constant : Constant  Value=3.594
  Constant1 : Constant  Value=3.594
  Cos : Trigonometry  Operator=cos
  Magnitude Squared1 : Math  Operator=magnitude^2
  Product5 : Product
  Product6 : Product
  Sin : Trigonometry
  Square Root1 : Sqrt
  Subtract : Sum  Inputs=+-
  Switch : Switch  SaturateOnIntegerOverflow=off  InputSameDT=off
  thrust curve N5800 : Lookup_n-D  NumberOfTableDimensions=1  BreakpointsForDimension1=|  BreakpointsForDimension2=[1:3]  Table=|  InternalRulePriority=Speed  RndMeth=Simplest
      BreakpointsForDimension1=|
      | [0.019
      | 0.049
      | 0.103
      | 0.384
      | 1.109
      | 1.569
      | 1.991
      | 2.622
      | 3.011
      | 3.192
      | 3.334
      | 3.423
      | 3.513
      | 3.581
      | 3.594]
      Table=|
      | [6694.9
      | 6720.292
      | 6593.334
      | 6677.973
      | 6957.279
      | 6940.352
      | 6720.292
      | 6009.329
      | 3275.507
      | 2606.864
      | 1599.666
      | 1041.053
      | 389.337
      | 220.06
      | 0.0]
  horizontal thrust : Outport
  vertical thrust : Outport  Port=2
  magnitude of T : Outport  Port=3
  wires:
  Clock/1 -> Switch/1, Subtract/2
  thrust curve N5800/1 -> Product6/1, Product5/1, magnitude of T/1
  Cos/1 -> Product5/2
  Sin/1 -> Product6/2
  pitch angle/1 -> Sin/1, Cos/1
  Product5/1 -> Magnitude Squared1/1
  Subtract/1 -> Switch/2
  Constant/1 -> Subtract/1
  Switch/1 -> thrust curve N5800/1
  Constant1/1 -> Switch/3
  Product6/1 -> horizontal thrust/1
  Magnitude Squared1/1 -> Square Root1/1
  Square Root1/1 -> vertical thrust/1

== matlab function ver1_3DOF_draft2/drag/drag curve function ==
  data: x input; z output; y input
function z = fcn(x, y)
%x is extension, y is mach number 
z = -24.372 - 388.42*x + 141.45*y + 43483*x^2 - 668.50*x*y - 153.02*y^2 - 1126600*x^3 + 4575.4*x^2*y + 3358.9*x*y^2 + 132.22*y^3;

== matlab function ver1_3DOF_draft2/drag/drag curve function1 ==
  data: x input; z output; y input
function z = fcn(x, y)
%x is extension, y is mach number 
z = -24.372 - 388.42*x + 141.45*y + 43483*x^2 - 668.50*x*y - 153.02*y^2 - 1126600*x^3 + 4575.4*x^2*y + 3358.9*x*y^2 + 132.22*y^3;
